simulink model "EarlyReturn16"  (R2020b)
settings: Solver=VariableStepAuto  StartTime=0.0  StopTime=0.1  RelTol=1e-3
settings Model: Creator=BEAR  LastModifiedBy=apple
settings DataIOCC: ReturnWorkspaceOutputs=off
settings DebuggingCC: ArithmeticOperatorsInVariantConditions=warning
settings SFSimCC: SimUseLocalCustomCode=off  CustomCodeUndefinedFunction=UseInterfaceOnly
settings RTWCC: RTWUseLocalCustomCode=off

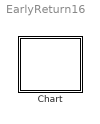
== system EarlyReturn16 ==
  Chart : Stateflow chart  TreatAsAtomicUnit=on

== stateflow chart EarlyReturn16/Chart ==
  state A
    en: fprintf("en_A")
    ex: fprintf("ex_A")
    state A1
      en: fprintf("en_A1")
      ex: fprintf("ex_A1")
    state A4
      en: fprintf("en_A4")
      ex: fprintf("ex_A4")
    state A3
      en: fprintf("en_A3")
    state A2
      en: fprintf("en_A2")
      ex: fprintf("ex_A2")
    (default) -> A1 : {x=1;}
    A1 -> A2 [order 3]
    A1 -> (junction 12) [order 2] : [x>0]{fprintf("outA1")}
    A1 -> A3 [order 1] : E[x>0]
    (junction 12) -> A4 : {E;fprintf("E")}
    A2 -> (junction 12) [order 2] : [x<0]{fprintf("outA2")}
    A2 -> A3 [order 1] : E[x<0]
  (default) -> A
  data: x local
  events: E local FUNCTION_CALL_EVENT
